simulink model "stateReduceOBS"  (Simulink 7.4)
settings: Solver=ode4  StartTime=0.0  StopTime=inf  FixedStep=0.01  RelTol=1e-3
undefined symbols (not defined in the file): aarm, apind, Aro, Bro, Cro, Dro, F, Fi, Lro
libraries: xpcnilib x2, simulink x1
settings Model: Creator=Skov  LastModifiedBy=Skov  SimulationMode=external  BufferReuse=off
settings DataIOCC: SaveState=on  InspectSignalLogs=on
settings OptimizationCC: BlockReduction=off  OptimizeBlockIOStorage=off  BufferReuse=off  ExpressionFolding=off  LocalBlockOutputs=off
settings HardwareCC: ProdIntDivRoundTo=Zero  ProdEndianess=LittleEndian  ProdHWDeviceType=Generic->32-bit x86 compatible
settings RTWCC: SystemTargetFile=xpctarget.tlc  TemplateMakefile=xpc_default_tmf  Description=xPC Target  ProcessScript=xpctarget_make_rtw_hook  RTWCompilerOptimization=On
settings xpcTargetCC: TargetFcnLib=ansi_tfl_table_tmw.mat  TargetFunctionLibrary=ANSI_C  ParMdlRefBuildCompliant=off  PortableWordSizes=off  xPCLoadParamSetFile=off

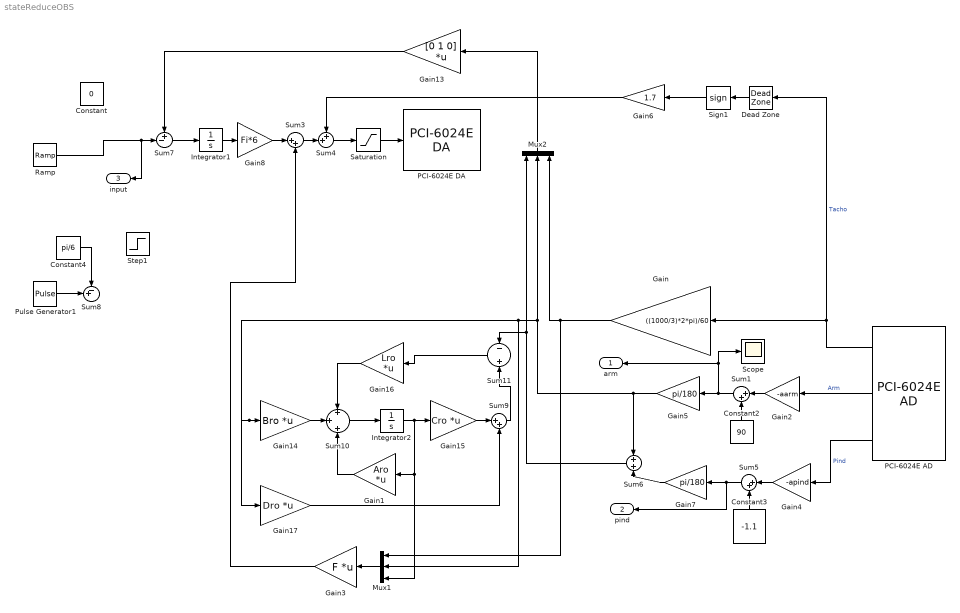
== system stateReduceOBS ==
  Constant : Constant  Value=0  OutDataType=fixdt(1, 16)  OutScaling=2^0
  Constant2 : Constant  Value=90  OutDataType=fixdt(1, 16)  OutScaling=2^0
  Constant3 : Constant  Value=-1.1  OutDataType=fixdt(1, 16)  OutScaling=2^0
  Constant4 : Constant  Value=pi/6  OutDataType=fixdt(1, 16)  OutScaling=2^0
  Dead Zone : DeadZone  LowerValue=-0.01  UpperValue=0.01  SaturateOnIntegerOverflow=on
  Gain : Gain  Gain=((1000/3)*2*pi)/60  ParameterDataType=fixdt(1, 16)  ParameterScaling=2^0  OutDataType=fixdt(1, 16)  OutScaling=2^0
  Gain1 : Gain  Gain=Aro  Multiplication=Matrix(K*u)  ParameterDataType=fixdt(1, 16)  ParameterScaling=2^0  OutDataType=fixdt(1, 16)  OutScaling=2^0
  Gain13 : Gain  Gain=[0 1 0]  Multiplication=Matrix(K*u)  ParameterDataType=fixdt(1, 16)  ParameterScaling=2^0  OutDataType=fixdt(1, 16)  OutScaling=2^0
  Gain14 : Gain  Gain=Bro  Multiplication=Matrix(K*u)  ParameterDataType=fixdt(1, 16)  ParameterScaling=2^0  OutDataType=fixdt(1, 16)  OutScaling=2^0
  Gain15 : Gain  Gain=Cro  Multiplication=Matrix(K*u)  ParameterDataType=fixdt(1, 16)  ParameterScaling=2^0  OutDataType=fixdt(1, 16)  OutScaling=2^0
  Gain16 : Gain  Gain=Lro  Multiplication=Matrix(K*u)  ParameterDataType=fixdt(1, 16)  ParameterScaling=2^0  OutDataType=fixdt(1, 16)  OutScaling=2^0
  Gain17 : Gain  Gain=Dro  Multiplication=Matrix(K*u)  ParameterDataType=fixdt(1, 16)  ParameterScaling=2^0  OutDataType=fixdt(1, 16)  OutScaling=2^0
  Gain2 : Gain  Gain=-aarm  ParameterDataType=fixdt(1, 16)  ParameterScaling=2^0  OutDataType=fixdt(1, 16)  OutScaling=2^0
  Gain3 : Gain  Gain=F  Multiplication=Matrix(K*u)  ParameterDataType=fixdt(1, 16)  ParameterScaling=2^0  OutDataType=fixdt(1, 16)  OutScaling=2^0
  Gain4 : Gain  Gain=-apind  ParameterDataType=fixdt(1, 16)  ParameterScaling=2^0  OutDataType=fixdt(1, 16)  OutScaling=2^0
  Gain5 : Gain  Gain=pi/180  ParameterDataType=fixdt(1, 16)  ParameterScaling=2^0  OutDataType=fixdt(1, 16)  OutScaling=2^0
  Gain6 : Gain  Gain=1.7  ParameterDataType=fixdt(1, 16)  ParameterScaling=2^0  OutDataType=fixdt(1, 16)  OutScaling=2^0
  Gain7 : Gain  Gain=pi/180  ParameterDataType=fixdt(1, 16)  ParameterScaling=2^0  OutDataType=fixdt(1, 16)  OutScaling=2^0
  Gain8 : Gain  Gain=Fi*6  ParameterDataType=fixdt(1, 16)  ParameterScaling=2^0  OutDataType=fixdt(1, 16)  OutScaling=2^0
  Integrator1 : Integrator  InitialCondition=[0]
  Integrator2 : Integrator  InitialCondition=[0 0]
  Mux1 : Mux  Inputs=3
  Mux2 : Mux  Inputs=3
  PCI-6024E AD : xpcnilib/A//D/E Series/PCI-6024E AD  channel=[3 1 2]  range=[-10]  coupling=[0]  sampletime=0.01  slot=-1
  PCI-6024E DA : xpcnilib/D//A/E Series/PCI-6024E DA  channel=[1]  reset=[1]  initValue=[0]  sampletime=0.01  slot=-1
  Pulse Generator1 : DiscretePulseGenerator  PulseType=Time based  Amplitude=pi/3  Period=45  PulseWidth=50  PhaseDelay=0  SampleTime=1
  Ramp : simulink/Sources/Ramp  SystemSampleTime=-1  slope=pi/360  start=10  X0=0
  Saturation : Saturate  UpperLimit=10  LowerLimit=-10  OutDataType=fixdt(1, 16)  OutScaling=2^0
  Scope : Scope
      settings: YMin=-25  YMax=22.5
  Sign1 : Signum
  Step1 : Step  After=0  SampleTime=0
  Sum{1,3,5,9} (4 alike) : Sum  Inputs=|++  OutDataType=fixdt(1, 16)  OutScaling=2^0
  Sum10 : Sum  Inputs=+|+|+  OutDataType=fixdt(1, 16)  OutScaling=2^0
  Sum11 : Sum  Inputs=-|+  OutDataType=fixdt(1, 16)  OutScaling=2^0
  Sum4 : Sum  Inputs=++|  OutDataType=fixdt(1, 16)  OutScaling=2^0
  Sum6 : Sum  Inputs=+|+  OutDataType=fixdt(1, 16)  OutScaling=2^0
  Sum7 : Sum  Inputs=+-|  OutDataType=fixdt(1, 16)  OutScaling=2^0
  Sum8 : Sum  Inputs=-+|  OutDataType=fixdt(1, 16)  OutScaling=2^0
  arm : Outport  OutDataType=fixdt(1, 16)  OutScaling=2^0
  pind : Outport  Port=2  OutDataType=fixdt(1, 16)  OutScaling=2^0
  input : Outport  Port=3  OutDataType=fixdt(1, 16)  OutScaling=2^0
  wires:
  Gain2/1 -> Sum1/1
  Constant2/1 -> Sum1/2
  Sum1/1 -> Gain5/1, Scope/1, arm/1
  PCI-6024E AD/1 -> Gain/1, Dead Zone/1  "Tacho"
  PCI-6024E AD/2 -> Gain2/1  "Arm"
  PCI-6024E AD/3 -> Gain4/1  "Pind"
  Gain4/1 -> Sum5/1
  Constant3/1 -> Sum5/2
  Sum5/1 -> Gain7/1, pind/1
  Gain13/1 -> Sum7/1
  Gain5/1 -> Sum6/1, Gain14/1, Gain17/1, Mux1/2, Mux2/2
  Gain/1 -> Mux1/1, Mux2/3
  Gain7/1 -> Sum6/2
  Dead Zone/1 -> Sign1/1
  Sign1/1 -> Gain6/1
  Gain6/1 -> Sum4/1
  Saturation/1 -> PCI-6024E DA/1
  Integrator2/1 -> Gain15/1, Gain1/1, Mux1/3
  Sum10/1 -> Integrator2/1
  Gain1/1 -> Sum10/3
  Gain14/1 -> Sum10/2
  Sum11/1 -> Gain16/1
  Gain3/1 -> Sum3/2
  Gain16/1 -> Sum10/1
  Mux1/1 -> Gain3/1
  Gain15/1 -> Sum9/1
  Sum9/1 -> Sum11/2
  Gain17/1 -> Sum9/2
  Sum6/1 -> Sum11/1, Mux2/1
  Mux2/1 -> Gain13/1
  Sum3/1 -> Sum4/2
  Integrator1/1 -> Gain8/1
  Gain8/1 -> Sum3/1
  Sum4/1 -> Saturation/1
  Sum7/1 -> Integrator1/1
  Constant4/1 -> Sum8/1
  Pulse Generator1/1 -> Sum8/2
  Ramp/1 -> Sum7/2, input/1
